simulink model "simlink_fcn"  (R2022b)
settings: Solver=VariableStepAuto  StartTime=0.0  StopTime=10.0  RelTol=1e-3
libraries: visionsources x1
settings Model: Creator=DSP-27  LastModifiedBy=DSP-27

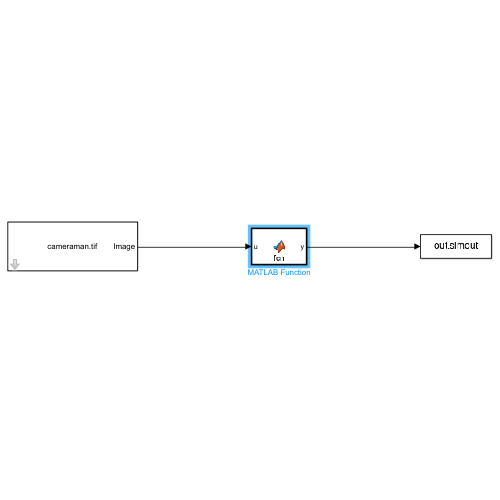
[thumbnail: Simulink's stored preview of the top-level diagram]
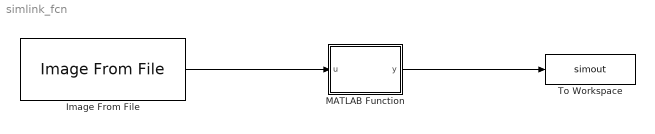
== system simlink_fcn ==
  Image From File : visionsources/Image From File  Tag=vipblks_nd  FileName=C:\Users\DSP-27\Downloads\cameraman.tif  Ts=inf  imagePorts=One multidimensional signal  OutPortLabels=R|G|B  ImageDataType=Inherit from input image  sdImageDataType=uint(8)  Signed=on  WordLength=16  FractionLengthMode=User-defined  FractionLength=15
  MATLAB Function : MATLAB Function  TreatAsAtomicUnit=on
  To Workspace : ToWorkspace  VariableName=simout  SampleTime=-1
      settings: Save2DSignal=2-D array (concatenate along first dimension)
  wires:
  Image From File/1 -> MATLAB Function/1(u)
  MATLAB Function/1(y) -> To Workspace/1

== matlab function simlink_fcn/MATLAB Function ==
  data: u input; y output
function y = fcn(u)


Im = u;
[M,N] = size(Im);
coder.extrinsic('dct2');
coder.extrinsic('idct2');
dct_coeff = zeros(M,N);
dct_coeff = dct2(Im);
Z = zeros(M,N);
Z_out = zeros(M,N);

for i = 1:M
    for j = 1:N
        if(i<=M/2 && j<=N/2)
            Z(i,j) = dct_coeff(i,j);
        else 
            Z(i,j) = 0;
        end
    end
end

Z_out = idct2(Z);

y = Z_out;
